simulink model "TestingReadings_2023a"  (R2023a)
settings: Solver=VariableStepAuto  StartTime=0.0  StopTime=40  RelTol=1e-3
settings Model: Creator=Jakob  LastModifiedBy=Jakob

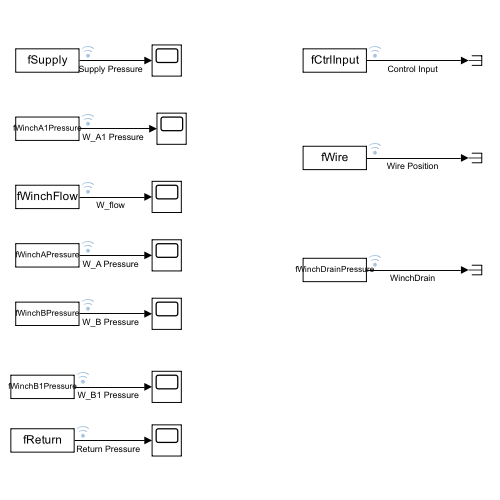
[thumbnail: Simulink's stored preview of the top-level diagram]
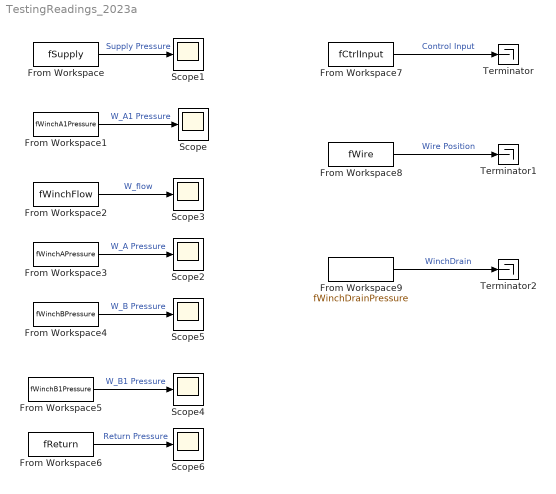
== system TestingReadings_2023a ==
  From Workspace : FromWorkspace  VariableName=fSupply  SampleTime=0.01
  From Workspace1 : FromWorkspace  VariableName=fWinchA1Pressure  SampleTime=0.01
  From Workspace2 : FromWorkspace  VariableName=fWinchFlow  SampleTime=0.01
  From Workspace3 : FromWorkspace  VariableName=fWinchAPressure  SampleTime=0.01
  From Workspace4 : FromWorkspace  VariableName=fWinchBPressure  SampleTime=0.01
  From Workspace5 : FromWorkspace  VariableName=fWinchB1Pressure  SampleTime=0.01
  From Workspace6 : FromWorkspace  VariableName=fReturn  SampleTime=0.01
  From Workspace7 : FromWorkspace  VariableName=fCtrlInput  SampleTime=0.01
  From Workspace8 : FromWorkspace  VariableName=fWire  SampleTime=0.01
  From Workspace9 : FromWorkspace  VariableName=fWinchDrainPressure  SampleTime=0.01
  Scope{,1..6} (7 alike) : Scope
  Terminator : Terminator
  Terminator1 : Terminator
  Terminator2 : Terminator
  wires:
  From Workspace1/1 -> Scope/1  "W_A1 Pressure"
  From Workspace/1 -> Scope1/1  "Supply Pressure"
  From Workspace2/1 -> Scope3/1  "W_flow"
  From Workspace3/1 -> Scope2/1  "W_A Pressure"
  From Workspace4/1 -> Scope5/1  "W_B Pressure"
  From Workspace5/1 -> Scope4/1  "W_B1 Pressure"
  From Workspace6/1 -> Scope6/1  "Return Pressure"
  From Workspace7/1 -> Terminator/1  "Control Input"
  From Workspace8/1 -> Terminator1/1  "Wire Position"
  From Workspace9/1 -> Terminator2/1  "WinchDrain"
